simulink model "gm_gm_mpu6050_interface"  (R2017a)
settings: Solver=FixedStepDiscrete  StartTime=0.0  StopTime=inf  RelTol=1e-3  EnableMultiTasking=on
PostLoadFcn:
  | ChipSelect = 1;  % choose I2C comms
  | AddressAlt  = 0;  % use default address
  | 
  | if AddressAlt == 1
  | % b1101001 (pin AD0 is logic high).
  | SlvAddr = uint8(bin2dec('1101001'));  % ADDR ALT = 1
  | else
  | % b1101000 (pin AD0 is logic low)
  | SlvAddr = uint8(bin2dec('1101000'));  % ADDR ALT = 0
  | end
  | 
  | % 0x3B 59 ACCEL_XOUT[15:8]
  | % 0x3C 60 ACCEL_XOUT[7:0]
  | % 0x3D 61 ACCEL_YOUT[15:8]
  | % 0x3E 62 ACCEL_YOUT[7:0]
  | % 0x3F 63 ACCEL_ZOUT[15:8]
  | % 0x40 64 ACCEL_ZOUT[7:0]
  | 
  | AccelXRegAddr = uint8(hex2dec('3B'));
  | AccelYRegAddr = uint8(hex2dec('3D'));
  | AccelZRegAddr = uint8(hex2dec('3F'));
  | 
  | % 0x43 67 GYRO_XOUT[15:8]
  | % 0x44 68 GYRO_XOUT[7:0]
  | % 0x45 69 GYRO_YOUT[15:8]
  | % 0x46 70 GYRO_YOUT[7:0]
  | % 0x47 71 GYRO_ZOUT[15:8]
  | % 0x48 72 GYRO_ZOUT[7:0]
  | 
  | GyroXRegAddr = uint8(hex2dec('43'));
  | GyroYRegAddr = uint8(hex2dec('45'));
  | GyroZRegAddr = uint8(hex2dec('47'));
  | 
  | deviceAddr = fi(SlvAddr,0,7,0);
  | 
  | powerRegAddr = uint8(hex2dec('6B'));
  | powerRegData = bin2dec('10000001');
undefined symbols (not defined in the file or in its folder): AXI4, codertarget, gcbh, Lite
libraries: axiinterfacelib x9
settings Model: Creator=skuznick  LastModifiedBy=Nicoe Welch
settings SolverCC: EnableConcurrentExecution=on  ConcurrentTasks=on  PositivePriorityOrder=on
settings DataIOCC: SaveOutput=off  SaveTime=off
settings OptimizationCC: BlockReduction=off  ConditionallyExecuteInputs=off  PassReuseOutputArgsAs=Individual arguments  MaxStackSize=64
settings DebuggingCC: AlgebraicLoopMsg=error  InheritedTsInSrcMsg=none  SingleTaskRateTransMsg=error  ParameterTunabilityLossMsg=error
settings HardwareCC: ProdBitPerPointer=32  ProdBitPerSizeT=32  ProdBitPerPtrDiffT=32  ProdLargestAtomicInteger=Long  ProdLargestAtomicFloat=Double  ProdWordSize=32  ProdHWDeviceType=ARM Compatible->ARM Cortex  TargetEndianess=LittleEndian
settings SFSimCC: MATLABDynamicMemAlloc=off
settings RTWCC: SystemTargetFile=ert.tlc  HardwareBoard=ZedBoard  TLCOptions="-aInlineSetEventsForThisBaseRateFcn=TLC_FALSE -aSuppressMultiTaskScheduler=TLC_FALSE  -aRateBasedStepFcn=0"  TemplateMakefile=ert_default_tmf  Description=Embedded Coder  GenerateReport=on  Toolchain=Xilinx Software Development Kit (SDK)  IncludeHyperlinkInReport=on  LaunchReport=on  GenerateTraceInfo=on  GenerateTraceReport=on  GenerateTraceReportSl=on  GenerateTraceReportSf=on  GenerateTraceReportEml=on
settings CodeAppCC: ForceParamTrailComments=on  IgnoreCustomStorageClasses=off  OperatorAnnotations=on  SimulinkDataObjDesc=on  SFDataObjDesc=on  MATLABFcnDesc=on  InsertBlockDesc=on  MATLABSourceComments=on

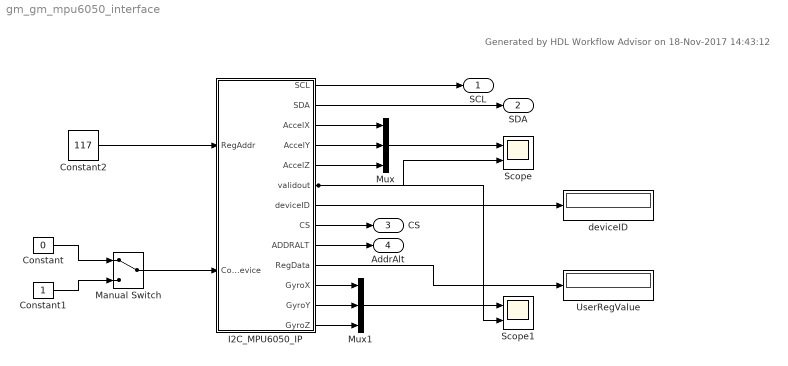
== system gm_gm_mpu6050_interface ==
  note: Generated by HDL Workflow Advisor on 18-Nov-2017 14:43:12
  Constant : Constant  Value=0  OutDataTypeStr=boolean  SampleTime=-1
  Constant1 : Constant  OutDataTypeStr=boolean  SampleTime=-1
  Constant2 : Constant  Value=117  OutDataTypeStr=uint8  SampleTime=-1
  I2C_MPU6050_IP : Subsystem  mask(AXI4-Lite/AXI4 Interface){}
      mask help:
      | This is an automatically generated subsystem block.
      | This contains the AXI interface blocks that communicate with the I2C_MPU60_ip IPCore generated from mpu6050/I2C_MPU6050_IP subsystem.
      mask Display: disp(sprintf('Xilinx Zynq \nAXI Interface'));
  Manual Switch : ManualSwitch
  Mux : Mux  Inputs=3
  Mux1 : Mux  Inputs=3
  Scope : Scope  NumInputPorts=2
  Scope1 : Scope  NumInputPorts=2
  UserRegValue : Display
  deviceID : Display
  SCL : Outport
  SDA : Outport  Port=2
  CS : Outport  Port=3
  AddrAlt : Outport  Port=4
  wires:
  I2C_MPU6050_IP/2(SDA) -> SDA/1
  I2C_MPU6050_IP/1(SCL) -> SCL/1
  I2C_MPU6050_IP/8(CS) -> CS/1
  I2C_MPU6050_IP/9(ADDRALT) -> AddrAlt/1
  I2C_MPU6050_IP/4(AccelY) -> Mux/2
  I2C_MPU6050_IP/3(AccelX) -> Mux/1
  I2C_MPU6050_IP/5(AccelZ) -> Mux/3
  I2C_MPU6050_IP/7(deviceID) -> deviceID/1
  I2C_MPU6050_IP/10(RegData) -> UserRegValue/1
  Mux/1 -> Scope/1
  Constant/1 -> Manual Switch/1
  Constant1/1 -> Manual Switch/2
  Manual Switch/1 -> I2C_MPU6050_IP/2(ConfigDevice)
  Constant2/1 -> I2C_MPU6050_IP/1(RegAddr)
  Mux1/1 -> Scope1/1
  I2C_MPU6050_IP/13(GyroZ) -> Mux1/3
  I2C_MPU6050_IP/11(GyroX) -> Mux1/1
  I2C_MPU6050_IP/12(GyroY) -> Mux1/2
  I2C_MPU6050_IP/6(validout) -> Scope/2, Scope1/2

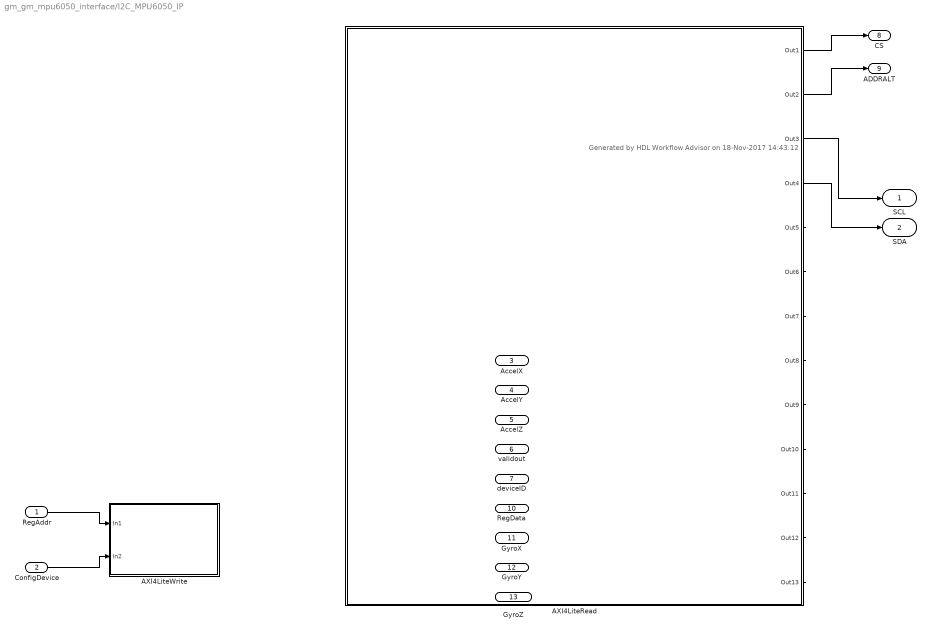
== system gm_gm_mpu6050_interface/I2C_MPU6050_IP ==
  note: Generated by HDL Workflow Advisor on 18-Nov-2017 14:43:12
  RegAddr : Inport  OutDataTypeStr=uint8  SampleTime=0.2
  ConfigDevice : Inport  Port=2  OutDataTypeStr=boolean  SampleTime=0.2
  AXI4LiteRead : Subsystem
  AXI4LiteWrite : Subsystem
  SCL : Outport
  SDA : Outport  Port=2
  AccelX : Outport  Port=3
  AccelY : Outport  Port=4
  AccelZ : Outport  Port=5
  validout : Outport  Port=6
  deviceID : Outport  Port=7
  CS : Outport  Port=8
  ADDRALT : Outport  Port=9
  RegData : Outport  Port=10
  GyroX : Outport  Port=11
  GyroY : Outport  Port=12
  GyroZ : Outport  Port=13
  wires:
  RegAddr/1 -> AXI4LiteWrite/1(In1)
  ConfigDevice/1 -> AXI4LiteWrite/2(In2)
  AXI4LiteRead/1(Out1) -> CS/1
  AXI4LiteRead/2(Out2) -> ADDRALT/1
  AXI4LiteRead/3(Out3) -> SCL/1
  AXI4LiteRead/4(Out4) -> SDA/1
  AXI4LiteRead/5(Out5) -> AccelX/1
  AXI4LiteRead/6(Out6) -> AccelY/1
  AXI4LiteRead/7(Out7) -> AccelZ/1
  AXI4LiteRead/8(Out8) -> validout/1
  AXI4LiteRead/9(Out9) -> deviceID/1
  AXI4LiteRead/10(Out10) -> RegData/1
  AXI4LiteRead/11(Out11) -> GyroX/1
  AXI4LiteRead/12(Out12) -> GyroY/1
  AXI4LiteRead/13(Out13) -> GyroZ/1

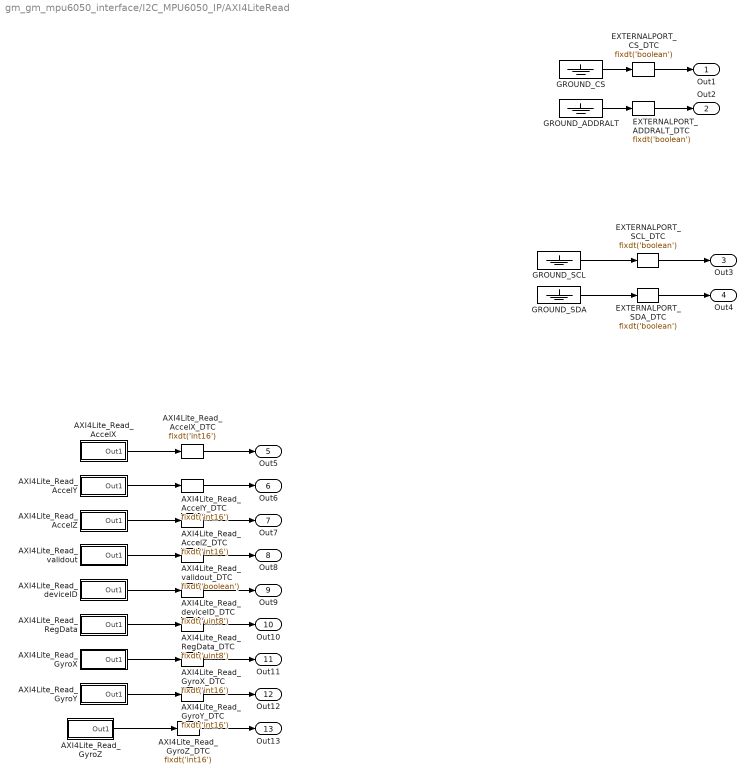
== system gm_gm_mpu6050_interface/I2C_MPU6050_IP/AXI4LiteRead ==
  AXI4Lite_Read_AccelX : Subsystem  InitFcn=codertarget.zynq.internal.registerAXIInterfaceBlocks(gcbh);  mask(AXI4-Interface Read){AXIInterfaceType='AXI4-Lite', DeviceName='/dev/mwipcore', RegisterOffset=hex2dec('104'), DataLength=1, DataType='uint32', SampleTime=-1, blockPlatform=ZYNQ, SimulateUsing=Interpreted Execution}
      mask prompts: AXIInterfaceType "AXI interface:"; DeviceName "Device name:"; RegisterOffset "Register offset:"; DataLength "Output vector size:"; DataType "Data type:"; SampleTime "Sample time:"; blockPlatform "Block Platform:"; SimulateUsing "Simulate Using:"
      mask help:
      | Read data from the IP core device using AXI interface.
      |
      | Set AXI interface parameter to 'AXI4-Lite' to read scalar data from the IP core register.
      |
      | Set AXI interface parameter to  'AXI4-Stream' to read vector data from DMA buffer. Use the Output vector size parameter to determine the number of samples read for each DMA transfer.
      mask init:
      | set_param(gcb, 'MaskDescription', DAStudio.message('zynq:utils:AXIReadMaskDisplay'));
      | set_param(gcb, 'MaskType','AXI4-Interface Read');
      | set_param(gcb, 'MaskHelp','eval(''slhelp([gcb,''''/AXI4-Interface Read''''])'');');
      | set_param(gcb, 'InitFcn', 'codertarget.zynq.internal.registerAXIInterfaceBlocks(gcbh);');
      mask Help: eval('slhelp([gcb,''/AXI4-Interface Read''])');
      mask Callback AXIInterfaceType:
      | if strcmpi(get_param(gcb, 'AXIInterfaceType'),'AXI4-Stream')
      |     set_param(gcb, 'MaskVisibilities',...
      |         {'on';'on';'off';'on';'on';'on';'off';'off'});
      | else
      |     set_param(gcb, 'MaskVisibilities',...
      |         {'on';'on';'on';'on';'on';'on';'off';'off'});
      | end
      mask TypeOptions SimulateUsing: Interpreted Execution | Code Generation
      mask Display:
      | text(0.50, 0.50, get_param([gcb,'/AXI4-Interface Read'], 'AXIInterfaceType'), ...
      |     'horizontalAlignment', 'center');
      | color('blue');
      | text(0.97, 0.87, get_param(gcb,'blockPlatform'), 'horizontalAlignment', 'right');
  AXI4Lite_Read_AccelX_DTC : DataTypeConversion  OutDataTypeStr=fixdt('int16')  ConvertRealWorld=Stored Integer (SI)
  AXI4Lite_Read_AccelY : Subsystem  InitFcn=codertarget.zynq.internal.registerAXIInterfaceBlocks(gcbh);  mask(AXI4-Interface Read){AXIInterfaceType='AXI4-Lite', DeviceName='/dev/mwipcore', RegisterOffset=hex2dec('108'), DataLength=1, DataType='uint32', SampleTime=-1, blockPlatform=ZYNQ, SimulateUsing=Interpreted Execution}
      mask prompts: AXIInterfaceType "AXI interface:"; DeviceName "Device name:"; RegisterOffset "Register offset:"; DataLength "Output vector size:"; DataType "Data type:"; SampleTime "Sample time:"; blockPlatform "Block Platform:"; SimulateUsing "Simulate Using:"
      mask help:
      | Read data from the IP core device using AXI interface.
      |
      | Set AXI interface parameter to 'AXI4-Lite' to read scalar data from the IP core register.
      |
      | Set AXI interface parameter to  'AXI4-Stream' to read vector data from DMA buffer. Use the Output vector size parameter to determine the number of samples read for each DMA transfer.
      mask init: same as gm_gm_mpu6050_interface/I2C_MPU6050_IP/AXI4LiteRead/AXI4Lite_Read_AccelX
      mask Help: eval('slhelp([gcb,''/AXI4-Interface Read''])');
      mask Callback AXIInterfaceType:
      | if strcmpi(get_param(gcb, 'AXIInterfaceType'),'AXI4-Stream')
      |     set_param(gcb, 'MaskVisibilities',...
      |         {'on';'on';'off';'on';'on';'on';'off';'off'});
      | else
      |     set_param(gcb, 'MaskVisibilities',...
      |         {'on';'on';'on';'on';'on';'on';'off';'off'});
      | end
      mask TypeOptions SimulateUsing: Interpreted Execution | Code Generation
      mask Display:
      | text(0.50, 0.50, get_param([gcb,'/AXI4-Interface Read'], 'AXIInterfaceType'), ...
      |     'horizontalAlignment', 'center');
      | color('blue');
      | text(0.97, 0.87, get_param(gcb,'blockPlatform'), 'horizontalAlignment', 'right');
  AXI4Lite_Read_AccelY_DTC : DataTypeConversion  OutDataTypeStr=fixdt('int16')  ConvertRealWorld=Stored Integer (SI)
  AXI4Lite_Read_AccelZ : Subsystem  InitFcn=codertarget.zynq.internal.registerAXIInterfaceBlocks(gcbh);  mask(AXI4-Interface Read){AXIInterfaceType='AXI4-Lite', DeviceName='/dev/mwipcore', RegisterOffset=hex2dec('10C'), DataLength=1, DataType='uint32', SampleTime=-1, blockPlatform=ZYNQ, SimulateUsing=Interpreted Execution}
      mask prompts: AXIInterfaceType "AXI interface:"; DeviceName "Device name:"; RegisterOffset "Register offset:"; DataLength "Output vector size:"; DataType "Data type:"; SampleTime "Sample time:"; blockPlatform "Block Platform:"; SimulateUsing "Simulate Using:"
      mask help:
      | Read data from the IP core device using AXI interface.
      |
      | Set AXI interface parameter to 'AXI4-Lite' to read scalar data from the IP core register.
      |
      | Set AXI interface parameter to  'AXI4-Stream' to read vector data from DMA buffer. Use the Output vector size parameter to determine the number of samples read for each DMA transfer.
      mask init: same as gm_gm_mpu6050_interface/I2C_MPU6050_IP/AXI4LiteRead/AXI4Lite_Read_AccelX
      mask Help: eval('slhelp([gcb,''/AXI4-Interface Read''])');
      mask Callback AXIInterfaceType:
      | if strcmpi(get_param(gcb, 'AXIInterfaceType'),'AXI4-Stream')
      |     set_param(gcb, 'MaskVisibilities',...
      |         {'on';'on';'off';'on';'on';'on';'off';'off'});
      | else
      |     set_param(gcb, 'MaskVisibilities',...
      |         {'on';'on';'on';'on';'on';'on';'off';'off'});
      | end
      mask TypeOptions SimulateUsing: Interpreted Execution | Code Generation
      mask Display:
      | text(0.50, 0.50, get_param([gcb,'/AXI4-Interface Read'], 'AXIInterfaceType'), ...
      |     'horizontalAlignment', 'center');
      | color('blue');
      | text(0.97, 0.87, get_param(gcb,'blockPlatform'), 'horizontalAlignment', 'right');
  AXI4Lite_Read_AccelZ_DTC : DataTypeConversion  OutDataTypeStr=fixdt('int16')  ConvertRealWorld=Stored Integer (SI)
  AXI4Lite_Read_GyroX : Subsystem  InitFcn=codertarget.zynq.internal.registerAXIInterfaceBlocks(gcbh);  mask(AXI4-Interface Read){AXIInterfaceType='AXI4-Lite', DeviceName='/dev/mwipcore', RegisterOffset=hex2dec('120'), DataLength=1, DataType='uint32', SampleTime=-1, blockPlatform=ZYNQ, SimulateUsing=Interpreted Execution}
      mask prompts: AXIInterfaceType "AXI interface:"; DeviceName "Device name:"; RegisterOffset "Register offset:"; DataLength "Output vector size:"; DataType "Data type:"; SampleTime "Sample time:"; blockPlatform "Block Platform:"; SimulateUsing "Simulate Using:"
      mask help:
      | Read data from the IP core device using AXI interface.
      |
      | Set AXI interface parameter to 'AXI4-Lite' to read scalar data from the IP core register.
      |
      | Set AXI interface parameter to  'AXI4-Stream' to read vector data from DMA buffer. Use the Output vector size parameter to determine the number of samples read for each DMA transfer.
      mask init: same as gm_gm_mpu6050_interface/I2C_MPU6050_IP/AXI4LiteRead/AXI4Lite_Read_AccelX
      mask Help: eval('slhelp([gcb,''/AXI4-Interface Read''])');
      mask Callback AXIInterfaceType:
      | if strcmpi(get_param(gcb, 'AXIInterfaceType'),'AXI4-Stream')
      |     set_param(gcb, 'MaskVisibilities',...
      |         {'on';'on';'off';'on';'on';'on';'off';'off'});
      | else
      |     set_param(gcb, 'MaskVisibilities',...
      |         {'on';'on';'on';'on';'on';'on';'off';'off'});
      | end
      mask TypeOptions SimulateUsing: Interpreted Execution | Code Generation
      mask Display:
      | text(0.50, 0.50, get_param([gcb,'/AXI4-Interface Read'], 'AXIInterfaceType'), ...
      |     'horizontalAlignment', 'center');
      | color('blue');
      | text(0.97, 0.87, get_param(gcb,'blockPlatform'), 'horizontalAlignment', 'right');
  AXI4Lite_Read_GyroX_DTC : DataTypeConversion  OutDataTypeStr=fixdt('int16')  ConvertRealWorld=Stored Integer (SI)
  AXI4Lite_Read_GyroY : Subsystem  InitFcn=codertarget.zynq.internal.registerAXIInterfaceBlocks(gcbh);  mask(AXI4-Interface Read){AXIInterfaceType='AXI4-Lite', DeviceName='/dev/mwipcore', RegisterOffset=hex2dec('124'), DataLength=1, DataType='uint32', SampleTime=-1, blockPlatform=ZYNQ, SimulateUsing=Interpreted Execution}
      mask prompts: AXIInterfaceType "AXI interface:"; DeviceName "Device name:"; RegisterOffset "Register offset:"; DataLength "Output vector size:"; DataType "Data type:"; SampleTime "Sample time:"; blockPlatform "Block Platform:"; SimulateUsing "Simulate Using:"
      mask help:
      | Read data from the IP core device using AXI interface.
      |
      | Set AXI interface parameter to 'AXI4-Lite' to read scalar data from the IP core register.
      |
      | Set AXI interface parameter to  'AXI4-Stream' to read vector data from DMA buffer. Use the Output vector size parameter to determine the number of samples read for each DMA transfer.
      mask init: same as gm_gm_mpu6050_interface/I2C_MPU6050_IP/AXI4LiteRead/AXI4Lite_Read_AccelX
      mask Help: eval('slhelp([gcb,''/AXI4-Interface Read''])');
      mask Callback AXIInterfaceType:
      | if strcmpi(get_param(gcb, 'AXIInterfaceType'),'AXI4-Stream')
      |     set_param(gcb, 'MaskVisibilities',...
      |         {'on';'on';'off';'on';'on';'on';'off';'off'});
      | else
      |     set_param(gcb, 'MaskVisibilities',...
      |         {'on';'on';'on';'on';'on';'on';'off';'off'});
      | end
      mask TypeOptions SimulateUsing: Interpreted Execution | Code Generation
      mask Display:
      | text(0.50, 0.50, get_param([gcb,'/AXI4-Interface Read'], 'AXIInterfaceType'), ...
      |     'horizontalAlignment', 'center');
      | color('blue');
      | text(0.97, 0.87, get_param(gcb,'blockPlatform'), 'horizontalAlignment', 'right');
  AXI4Lite_Read_GyroY_DTC : DataTypeConversion  OutDataTypeStr=fixdt('int16')  ConvertRealWorld=Stored Integer (SI)
  AXI4Lite_Read_GyroZ : Subsystem  InitFcn=codertarget.zynq.internal.registerAXIInterfaceBlocks(gcbh);  mask(AXI4-Interface Read){AXIInterfaceType='AXI4-Lite', DeviceName='/dev/mwipcore', RegisterOffset=hex2dec('128'), DataLength=1, DataType='uint32', SampleTime=-1, blockPlatform=ZYNQ, SimulateUsing=Interpreted Execution}
      mask prompts: AXIInterfaceType "AXI interface:"; DeviceName "Device name:"; RegisterOffset "Register offset:"; DataLength "Output vector size:"; DataType "Data type:"; SampleTime "Sample time:"; blockPlatform "Block Platform:"; SimulateUsing "Simulate Using:"
      mask help:
      | Read data from the IP core device using AXI interface.
      |
      | Set AXI interface parameter to 'AXI4-Lite' to read scalar data from the IP core register.
      |
      | Set AXI interface parameter to  'AXI4-Stream' to read vector data from DMA buffer. Use the Output vector size parameter to determine the number of samples read for each DMA transfer.
      mask init: same as gm_gm_mpu6050_interface/I2C_MPU6050_IP/AXI4LiteRead/AXI4Lite_Read_AccelX
      mask Help: eval('slhelp([gcb,''/AXI4-Interface Read''])');
      mask Callback AXIInterfaceType:
      | if strcmpi(get_param(gcb, 'AXIInterfaceType'),'AXI4-Stream')
      |     set_param(gcb, 'MaskVisibilities',...
      |         {'on';'on';'off';'on';'on';'on';'off';'off'});
      | else
      |     set_param(gcb, 'MaskVisibilities',...
      |         {'on';'on';'on';'on';'on';'on';'off';'off'});
      | end
      mask TypeOptions SimulateUsing: Interpreted Execution | Code Generation
      mask Display:
      | text(0.50, 0.50, get_param([gcb,'/AXI4-Interface Read'], 'AXIInterfaceType'), ...
      |     'horizontalAlignment', 'center');
      | color('blue');
      | text(0.97, 0.87, get_param(gcb,'blockPlatform'), 'horizontalAlignment', 'right');
  AXI4Lite_Read_GyroZ_DTC : DataTypeConversion  OutDataTypeStr=fixdt('int16')  ConvertRealWorld=Stored Integer (SI)
  AXI4Lite_Read_RegData : Subsystem  InitFcn=codertarget.zynq.internal.registerAXIInterfaceBlocks(gcbh);  mask(AXI4-Interface Read){AXIInterfaceType='AXI4-Lite', DeviceName='/dev/mwipcore', RegisterOffset=hex2dec('11C'), DataLength=1, DataType='uint32', SampleTime=-1, blockPlatform=ZYNQ, SimulateUsing=Interpreted Execution}
      mask prompts: AXIInterfaceType "AXI interface:"; DeviceName "Device name:"; RegisterOffset "Register offset:"; DataLength "Output vector size:"; DataType "Data type:"; SampleTime "Sample time:"; blockPlatform "Block Platform:"; SimulateUsing "Simulate Using:"
      mask help:
      | Read data from the IP core device using AXI interface.
      |
      | Set AXI interface parameter to 'AXI4-Lite' to read scalar data from the IP core register.
      |
      | Set AXI interface parameter to  'AXI4-Stream' to read vector data from DMA buffer. Use the Output vector size parameter to determine the number of samples read for each DMA transfer.
      mask init: same as gm_gm_mpu6050_interface/I2C_MPU6050_IP/AXI4LiteRead/AXI4Lite_Read_AccelX
      mask Help: eval('slhelp([gcb,''/AXI4-Interface Read''])');
      mask Callback AXIInterfaceType:
      | if strcmpi(get_param(gcb, 'AXIInterfaceType'),'AXI4-Stream')
      |     set_param(gcb, 'MaskVisibilities',...
      |         {'on';'on';'off';'on';'on';'on';'off';'off'});
      | else
      |     set_param(gcb, 'MaskVisibilities',...
      |         {'on';'on';'on';'on';'on';'on';'off';'off'});
      | end
      mask TypeOptions SimulateUsing: Interpreted Execution | Code Generation
      mask Display:
      | text(0.50, 0.50, get_param([gcb,'/AXI4-Interface Read'], 'AXIInterfaceType'), ...
      |     'horizontalAlignment', 'center');
      | color('blue');
      | text(0.97, 0.87, get_param(gcb,'blockPlatform'), 'horizontalAlignment', 'right');
  AXI4Lite_Read_RegData_DTC : DataTypeConversion  OutDataTypeStr=fixdt('uint8')  ConvertRealWorld=Stored Integer (SI)
  AXI4Lite_Read_deviceID : Subsystem  InitFcn=codertarget.zynq.internal.registerAXIInterfaceBlocks(gcbh);  mask(AXI4-Interface Read){AXIInterfaceType='AXI4-Lite', DeviceName='/dev/mwipcore', RegisterOffset=hex2dec('118'), DataLength=1, DataType='uint32', SampleTime=-1, blockPlatform=ZYNQ, SimulateUsing=Interpreted Execution}
      mask prompts: AXIInterfaceType "AXI interface:"; DeviceName "Device name:"; RegisterOffset "Register offset:"; DataLength "Output vector size:"; DataType "Data type:"; SampleTime "Sample time:"; blockPlatform "Block Platform:"; SimulateUsing "Simulate Using:"
      mask help:
      | Read data from the IP core device using AXI interface.
      |
      | Set AXI interface parameter to 'AXI4-Lite' to read scalar data from the IP core register.
      |
      | Set AXI interface parameter to  'AXI4-Stream' to read vector data from DMA buffer. Use the Output vector size parameter to determine the number of samples read for each DMA transfer.
      mask init: same as gm_gm_mpu6050_interface/I2C_MPU6050_IP/AXI4LiteRead/AXI4Lite_Read_AccelX
      mask Help: eval('slhelp([gcb,''/AXI4-Interface Read''])');
      mask Callback AXIInterfaceType:
      | if strcmpi(get_param(gcb, 'AXIInterfaceType'),'AXI4-Stream')
      |     set_param(gcb, 'MaskVisibilities',...
      |         {'on';'on';'off';'on';'on';'on';'off';'off'});
      | else
      |     set_param(gcb, 'MaskVisibilities',...
      |         {'on';'on';'on';'on';'on';'on';'off';'off'});
      | end
      mask TypeOptions SimulateUsing: Interpreted Execution | Code Generation
      mask Display:
      | text(0.50, 0.50, get_param([gcb,'/AXI4-Interface Read'], 'AXIInterfaceType'), ...
      |     'horizontalAlignment', 'center');
      | color('blue');
      | text(0.97, 0.87, get_param(gcb,'blockPlatform'), 'horizontalAlignment', 'right');
  AXI4Lite_Read_deviceID_DTC : DataTypeConversion  OutDataTypeStr=fixdt('uint8')  ConvertRealWorld=Stored Integer (SI)
  AXI4Lite_Read_validout : Subsystem  InitFcn=codertarget.zynq.internal.registerAXIInterfaceBlocks(gcbh);  mask(AXI4-Interface Read){AXIInterfaceType='AXI4-Lite', DeviceName='/dev/mwipcore', RegisterOffset=hex2dec('110'), DataLength=1, DataType='uint32', SampleTime=-1, blockPlatform=ZYNQ, SimulateUsing=Interpreted Execution}
      mask prompts: AXIInterfaceType "AXI interface:"; DeviceName "Device name:"; RegisterOffset "Register offset:"; DataLength "Output vector size:"; DataType "Data type:"; SampleTime "Sample time:"; blockPlatform "Block Platform:"; SimulateUsing "Simulate Using:"
      mask help:
      | Read data from the IP core device using AXI interface.
      |
      | Set AXI interface parameter to 'AXI4-Lite' to read scalar data from the IP core register.
      |
      | Set AXI interface parameter to  'AXI4-Stream' to read vector data from DMA buffer. Use the Output vector size parameter to determine the number of samples read for each DMA transfer.
      mask init: same as gm_gm_mpu6050_interface/I2C_MPU6050_IP/AXI4LiteRead/AXI4Lite_Read_AccelX
      mask Help: eval('slhelp([gcb,''/AXI4-Interface Read''])');
      mask Callback AXIInterfaceType:
      | if strcmpi(get_param(gcb, 'AXIInterfaceType'),'AXI4-Stream')
      |     set_param(gcb, 'MaskVisibilities',...
      |         {'on';'on';'off';'on';'on';'on';'off';'off'});
      | else
      |     set_param(gcb, 'MaskVisibilities',...
      |         {'on';'on';'on';'on';'on';'on';'off';'off'});
      | end
      mask TypeOptions SimulateUsing: Interpreted Execution | Code Generation
      mask Display:
      | text(0.50, 0.50, get_param([gcb,'/AXI4-Interface Read'], 'AXIInterfaceType'), ...
      |     'horizontalAlignment', 'center');
      | color('blue');
      | text(0.97, 0.87, get_param(gcb,'blockPlatform'), 'horizontalAlignment', 'right');
  AXI4Lite_Read_validout_DTC : DataTypeConversion  OutDataTypeStr=fixdt('boolean')  ConvertRealWorld=Stored Integer (SI)
  EXTERNALPORT_ADDRALT_DTC : DataTypeConversion  OutDataTypeStr=fixdt('boolean')
  EXTERNALPORT_CS_DTC : DataTypeConversion  OutDataTypeStr=fixdt('boolean')
  EXTERNALPORT_SCL_DTC : DataTypeConversion  OutDataTypeStr=fixdt('boolean')
  EXTERNALPORT_SDA_DTC : DataTypeConversion  OutDataTypeStr=fixdt('boolean')
  GROUND_ADDRALT : Ground
  GROUND_CS : Ground
  GROUND_SCL : Ground
  GROUND_SDA : Ground
  Out1 : Outport
  Out2 : Outport  Port=2
  Out3 : Outport  Port=3
  Out4 : Outport  Port=4
  Out5 : Outport  Port=5
  Out6 : Outport  Port=6
  Out7 : Outport  Port=7
  Out8 : Outport  Port=8
  Out9 : Outport  Port=9
  Out10 : Outport  Port=10
  Out11 : Outport  Port=11
  Out12 : Outport  Port=12
  Out13 : Outport  Port=13
  wires:
  AXI4Lite_Read_AccelX/1(Out1) -> AXI4Lite_Read_AccelX_DTC/1
  AXI4Lite_Read_AccelX_DTC/1 -> Out5/1
  AXI4Lite_Read_AccelY/1(Out1) -> AXI4Lite_Read_AccelY_DTC/1
  AXI4Lite_Read_AccelY_DTC/1 -> Out6/1
  AXI4Lite_Read_AccelZ/1(Out1) -> AXI4Lite_Read_AccelZ_DTC/1
  AXI4Lite_Read_AccelZ_DTC/1 -> Out7/1
  AXI4Lite_Read_GyroX/1(Out1) -> AXI4Lite_Read_GyroX_DTC/1
  AXI4Lite_Read_GyroX_DTC/1 -> Out11/1
  AXI4Lite_Read_GyroY/1(Out1) -> AXI4Lite_Read_GyroY_DTC/1
  AXI4Lite_Read_GyroY_DTC/1 -> Out12/1
  AXI4Lite_Read_GyroZ/1(Out1) -> AXI4Lite_Read_GyroZ_DTC/1
  AXI4Lite_Read_GyroZ_DTC/1 -> Out13/1
  AXI4Lite_Read_RegData/1(Out1) -> AXI4Lite_Read_RegData_DTC/1
  AXI4Lite_Read_RegData_DTC/1 -> Out10/1
  AXI4Lite_Read_deviceID/1(Out1) -> AXI4Lite_Read_deviceID_DTC/1
  AXI4Lite_Read_deviceID_DTC/1 -> Out9/1
  AXI4Lite_Read_validout/1(Out1) -> AXI4Lite_Read_validout_DTC/1
  AXI4Lite_Read_validout_DTC/1 -> Out8/1
  EXTERNALPORT_ADDRALT_DTC/1 -> Out2/1
  EXTERNALPORT_CS_DTC/1 -> Out1/1
  EXTERNALPORT_SCL_DTC/1 -> Out3/1
  EXTERNALPORT_SDA_DTC/1 -> Out4/1
  GROUND_ADDRALT/1 -> EXTERNALPORT_ADDRALT_DTC/1
  GROUND_CS/1 -> EXTERNALPORT_CS_DTC/1
  GROUND_SCL/1 -> EXTERNALPORT_SCL_DTC/1
  GROUND_SDA/1 -> EXTERNALPORT_SDA_DTC/1

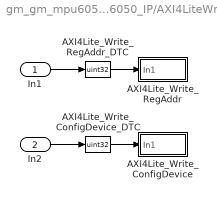
== system gm_gm_mpu6050_interface/I2C_MPU6050_IP/AXI4LiteWrite ==
  In1 : Inport  SampleTime=0.2
  In2 : Inport  Port=2  SampleTime=0.2
  AXI4Lite_Write_ConfigDevice : Subsystem  InitFcn=codertarget.zynq.internal.registerAXIInterfaceBlocks(gcbh);  mask(AXI4-Interface Write){AXIInterfaceType='AXI4-Lite', DeviceName='/dev/mwipcore', RegisterOffset=hex2dec('100'), blockPlatform=ZYNQ, SimulateUsing=Interpreted execution}
      mask prompts: AXIInterfaceType "AXI interface:"; DeviceName "Device name:"; RegisterOffset "Register offset:"; blockPlatform "Block platform:"; SimulateUsing "Simulate using:"
      mask help:
      | Write data to the IP core device using AXI interface.
      |
      | Set AXI interface parameter to 'AXI4-Lite' to write scalar data to the IP core register.
      |
      | Set AXI interface parameter to  'AXI4-Stream' to write vector data to DMA buffer.
      mask init:
      | set_param(gcb, 'MaskDescription', DAStudio.message('zynq:utils:AXIWriteMaskDisplay'));
      | set_param(gcb, 'MaskType','AXI4-Interface Write');
      | set_param(gcb, 'MaskHelp','eval(''slhelp([gcb,''''/AXI4-Interface Write''''])'');');
      | set_param(gcb, 'InitFcn', 'codertarget.zynq.internal.registerAXIInterfaceBlocks(gcbh);')
      mask Help: eval('slhelp([gcb,''/AXI4-Interface Write''])');
      mask Callback AXIInterfaceType:
      | if strcmpi(get_param(gcb, 'AXIInterfaceType'),'AXI4-Stream')
      |     set_param(gcb, 'MaskVisibilities',...
      |         {'on';'on';'off';'off';'off'});
      | else
      |     set_param(gcb, 'MaskVisibilities',...
      |         {'on';'on';'on';'off';'off'});
      | end
      mask TypeOptions SimulateUsing: Interpreted execution | Code generation
      mask Display:
      | text(0.50, 0.50, get_param([gcb,'/AXI4-Interface Write'], 'AXIInterfaceType'), ...
      |     'horizontalAlignment', 'center');
      | color('blue');
      | text(0.97, 0.87, get_param(gcb,'blockPlatform'), 'horizontalAlignment', 'right');
  AXI4Lite_Write_ConfigDevice_DTC : DataTypeConversion  OutDataTypeStr=uint32  ConvertRealWorld=Stored Integer (SI)
  AXI4Lite_Write_RegAddr : Subsystem  InitFcn=codertarget.zynq.internal.registerAXIInterfaceBlocks(gcbh);  mask(AXI4-Interface Write){AXIInterfaceType='AXI4-Lite', DeviceName='/dev/mwipcore', RegisterOffset=hex2dec('114'), blockPlatform=ZYNQ, SimulateUsing=Interpreted execution}
      mask prompts: AXIInterfaceType "AXI interface:"; DeviceName "Device name:"; RegisterOffset "Register offset:"; blockPlatform "Block platform:"; SimulateUsing "Simulate using:"
      mask help:
      | Write data to the IP core device using AXI interface.
      |
      | Set AXI interface parameter to 'AXI4-Lite' to write scalar data to the IP core register.
      |
      | Set AXI interface parameter to  'AXI4-Stream' to write vector data to DMA buffer.
      mask init: same as gm_gm_mpu6050_interface/I2C_MPU6050_IP/AXI4LiteWrite/AXI4Lite_Write_ConfigDevice
      mask Help: eval('slhelp([gcb,''/AXI4-Interface Write''])');
      mask Callback AXIInterfaceType:
      | if strcmpi(get_param(gcb, 'AXIInterfaceType'),'AXI4-Stream')
      |     set_param(gcb, 'MaskVisibilities',...
      |         {'on';'on';'off';'off';'off'});
      | else
      |     set_param(gcb, 'MaskVisibilities',...
      |         {'on';'on';'on';'off';'off'});
      | end
      mask TypeOptions SimulateUsing: Interpreted execution | Code generation
      mask Display:
      | text(0.50, 0.50, get_param([gcb,'/AXI4-Interface Write'], 'AXIInterfaceType'), ...
      |     'horizontalAlignment', 'center');
      | color('blue');
      | text(0.97, 0.87, get_param(gcb,'blockPlatform'), 'horizontalAlignment', 'right');
  AXI4Lite_Write_RegAddr_DTC : DataTypeConversion  OutDataTypeStr=uint32  ConvertRealWorld=Stored Integer (SI)
  wires:
  In1/1 -> AXI4Lite_Write_RegAddr_DTC/1
  In2/1 -> AXI4Lite_Write_ConfigDevice_DTC/1
  AXI4Lite_Write_ConfigDevice_DTC/1 -> AXI4Lite_Write_ConfigDevice/1(In1)
  AXI4Lite_Write_RegAddr_DTC/1 -> AXI4Lite_Write_RegAddr/1(In1)

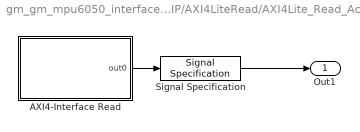
== system gm_gm_mpu6050_interface/I2C_MPU6050_IP/AXI4LiteRead/AXI4Lite_Read_AccelX ==
  AXI4-Interface Read : Subsystem
  Signal Specification : SignalSpecification
  Out1 : Outport
  wires:
  AXI4-Interface Read/1(out0) -> Signal Specification/1
  Signal Specification/1 -> Out1/1

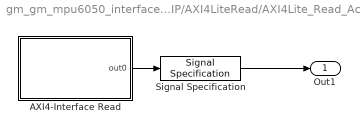
== system gm_gm_mpu6050_interface/I2C_MPU6050_IP/AXI4LiteRead/AXI4Lite_Read_AccelY ==
  AXI4-Interface Read : Subsystem
  Signal Specification : SignalSpecification
  Out1 : Outport
  wires:
  AXI4-Interface Read/1(out0) -> Signal Specification/1
  Signal Specification/1 -> Out1/1

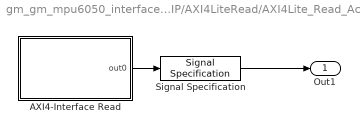
== system gm_gm_mpu6050_interface/I2C_MPU6050_IP/AXI4LiteRead/AXI4Lite_Read_AccelZ ==
  AXI4-Interface Read : Subsystem
  Signal Specification : SignalSpecification
  Out1 : Outport
  wires:
  AXI4-Interface Read/1(out0) -> Signal Specification/1
  Signal Specification/1 -> Out1/1

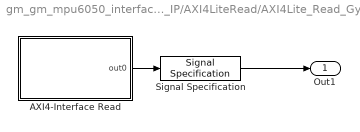
== system gm_gm_mpu6050_interface/I2C_MPU6050_IP/AXI4LiteRead/AXI4Lite_Read_GyroX ==
  AXI4-Interface Read : Subsystem
  Signal Specification : SignalSpecification
  Out1 : Outport
  wires:
  AXI4-Interface Read/1(out0) -> Signal Specification/1
  Signal Specification/1 -> Out1/1

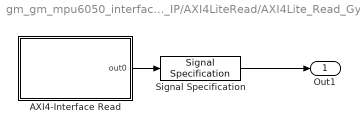
== system gm_gm_mpu6050_interface/I2C_MPU6050_IP/AXI4LiteRead/AXI4Lite_Read_GyroY ==
  AXI4-Interface Read : Subsystem
  Signal Specification : SignalSpecification
  Out1 : Outport
  wires:
  AXI4-Interface Read/1(out0) -> Signal Specification/1
  Signal Specification/1 -> Out1/1

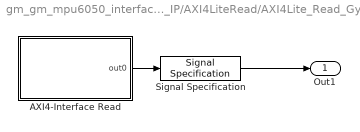
== system gm_gm_mpu6050_interface/I2C_MPU6050_IP/AXI4LiteRead/AXI4Lite_Read_GyroZ ==
  AXI4-Interface Read : Subsystem
  Signal Specification : SignalSpecification
  Out1 : Outport
  wires:
  AXI4-Interface Read/1(out0) -> Signal Specification/1
  Signal Specification/1 -> Out1/1

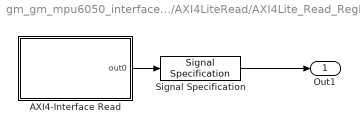
== system gm_gm_mpu6050_interface/I2C_MPU6050_IP/AXI4LiteRead/AXI4Lite_Read_RegData ==
  AXI4-Interface Read : Subsystem
  Signal Specification : SignalSpecification
  Out1 : Outport
  wires:
  AXI4-Interface Read/1(out0) -> Signal Specification/1
  Signal Specification/1 -> Out1/1

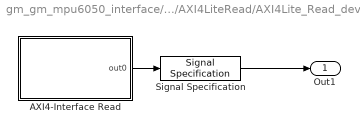
== system gm_gm_mpu6050_interface/I2C_MPU6050_IP/AXI4LiteRead/AXI4Lite_Read_deviceID ==
  AXI4-Interface Read : Subsystem
  Signal Specification : SignalSpecification
  Out1 : Outport
  wires:
  AXI4-Interface Read/1(out0) -> Signal Specification/1
  Signal Specification/1 -> Out1/1

== system gm_gm_mpu6050_interface/I2C_MPU6050_IP/AXI4LiteRead/AXI4Lite_Read_validout ==
  AXI4-Interface Read : Subsystem
  Signal Specification : SignalSpecification
  Out1 : Outport
  wires:
  AXI4-Interface Read/1(out0) -> Signal Specification/1
  Signal Specification/1 -> Out1/1

== system gm_gm_mpu6050_interface/I2C_MPU6050_IP/AXI4LiteWrite/AXI4Lite_Write_ConfigDevice ==
  In1 : Inport  OutDataTypeStr=uint32  SampleTime=0.2
  AXI4-Interface Write : Subsystem
  Signal Specification : SignalSpecification
  wires:
  In1/1 -> Signal Specification/1
  Signal Specification/1 -> AXI4-Interface Write/1(in0)

== system gm_gm_mpu6050_interface/I2C_MPU6050_IP/AXI4LiteWrite/AXI4Lite_Write_RegAddr ==
  In1 : Inport  OutDataTypeStr=uint32  SampleTime=0.2
  AXI4-Interface Write : Subsystem
  Signal Specification : SignalSpecification
  wires:
  In1/1 -> Signal Specification/1
  Signal Specification/1 -> AXI4-Interface Write/1(in0)

== system gm_gm_mpu6050_interface/I2C_MPU6050_IP/AXI4LiteRead/AXI4Lite_Read_AccelX/AXI4-Interface Read ==
  AXI4-Interface Read : axiinterfacelib/AXI4-Interface Read/AXI4-Interface Read  AXIInterfaceType=AXI4-Lite  DeviceName=/dev/mwipcore  RegisterOffset=RegisterOffset  DataType=uint32  DataLength=DataLength  SampleTime=SampleTime
      settings: SourceProductName=Embedded Coder Support Package for Xilinx Zynq-7000 Platform  SourceProductBaseCode=ECZYNQ7000
  out0 : Outport
  wires:
  AXI4-Interface Read/1 -> out0/1

== system gm_gm_mpu6050_interface/I2C_MPU6050_IP/AXI4LiteRead/AXI4Lite_Read_AccelY/AXI4-Interface Read ==
  AXI4-Interface Read : axiinterfacelib/AXI4-Interface Read/AXI4-Interface Read  AXIInterfaceType=AXI4-Lite  DeviceName=/dev/mwipcore  RegisterOffset=RegisterOffset  DataType=uint32  DataLength=DataLength  SampleTime=SampleTime
      settings: SourceProductName=Embedded Coder Support Package for Xilinx Zynq-7000 Platform  SourceProductBaseCode=ECZYNQ7000
  out0 : Outport
  wires:
  AXI4-Interface Read/1 -> out0/1

== system gm_gm_mpu6050_interface/I2C_MPU6050_IP/AXI4LiteRead/AXI4Lite_Read_AccelZ/AXI4-Interface Read ==
  AXI4-Interface Read : axiinterfacelib/AXI4-Interface Read/AXI4-Interface Read  AXIInterfaceType=AXI4-Lite  DeviceName=/dev/mwipcore  RegisterOffset=RegisterOffset  DataType=uint32  DataLength=DataLength  SampleTime=SampleTime
      settings: SourceProductName=Embedded Coder Support Package for Xilinx Zynq-7000 Platform  SourceProductBaseCode=ECZYNQ7000
  out0 : Outport
  wires:
  AXI4-Interface Read/1 -> out0/1

== system gm_gm_mpu6050_interface/I2C_MPU6050_IP/AXI4LiteRead/AXI4Lite_Read_GyroX/AXI4-Interface Read ==
  AXI4-Interface Read : axiinterfacelib/AXI4-Interface Read/AXI4-Interface Read  AXIInterfaceType=AXI4-Lite  DeviceName=/dev/mwipcore  RegisterOffset=RegisterOffset  DataType=uint32  DataLength=DataLength  SampleTime=SampleTime
      settings: SourceProductName=Embedded Coder Support Package for Xilinx Zynq-7000 Platform  SourceProductBaseCode=ECZYNQ7000
  out0 : Outport
  wires:
  AXI4-Interface Read/1 -> out0/1

== system gm_gm_mpu6050_interface/I2C_MPU6050_IP/AXI4LiteRead/AXI4Lite_Read_GyroY/AXI4-Interface Read ==
  AXI4-Interface Read : axiinterfacelib/AXI4-Interface Read/AXI4-Interface Read  AXIInterfaceType=AXI4-Lite  DeviceName=/dev/mwipcore  RegisterOffset=RegisterOffset  DataType=uint32  DataLength=DataLength  SampleTime=SampleTime
      settings: SourceProductName=Embedded Coder Support Package for Xilinx Zynq-7000 Platform  SourceProductBaseCode=ECZYNQ7000
  out0 : Outport
  wires:
  AXI4-Interface Read/1 -> out0/1

== system gm_gm_mpu6050_interface/I2C_MPU6050_IP/AXI4LiteRead/AXI4Lite_Read_GyroZ/AXI4-Interface Read ==
  AXI4-Interface Read : axiinterfacelib/AXI4-Interface Read/AXI4-Interface Read  AXIInterfaceType=AXI4-Lite  DeviceName=/dev/mwipcore  RegisterOffset=RegisterOffset  DataType=uint32  DataLength=DataLength  SampleTime=SampleTime
      settings: SourceProductName=Embedded Coder Support Package for Xilinx Zynq-7000 Platform  SourceProductBaseCode=ECZYNQ7000
  out0 : Outport
  wires:
  AXI4-Interface Read/1 -> out0/1

== system gm_gm_mpu6050_interface/I2C_MPU6050_IP/AXI4LiteRead/AXI4Lite_Read_RegData/AXI4-Interface Read ==
  AXI4-Interface Read : axiinterfacelib/AXI4-Interface Read/AXI4-Interface Read  AXIInterfaceType=AXI4-Lite  DeviceName=/dev/mwipcore  RegisterOffset=RegisterOffset  DataType=uint32  DataLength=DataLength  SampleTime=SampleTime
      settings: SourceProductName=Embedded Coder Support Package for Xilinx Zynq-7000 Platform  SourceProductBaseCode=ECZYNQ7000
  out0 : Outport
  wires:
  AXI4-Interface Read/1 -> out0/1

== system gm_gm_mpu6050_interface/I2C_MPU6050_IP/AXI4LiteRead/AXI4Lite_Read_deviceID/AXI4-Interface Read ==
  AXI4-Interface Read : axiinterfacelib/AXI4-Interface Read/AXI4-Interface Read  AXIInterfaceType=AXI4-Lite  DeviceName=/dev/mwipcore  RegisterOffset=RegisterOffset  DataType=uint32  DataLength=DataLength  SampleTime=SampleTime
      settings: SourceProductName=Embedded Coder Support Package for Xilinx Zynq-7000 Platform  SourceProductBaseCode=ECZYNQ7000
  out0 : Outport
  wires:
  AXI4-Interface Read/1 -> out0/1

== system gm_gm_mpu6050_interface/I2C_MPU6050_IP/AXI4LiteRead/AXI4Lite_Read_validout/AXI4-Interface Read ==
  AXI4-Interface Read : axiinterfacelib/AXI4-Interface Read/AXI4-Interface Read  AXIInterfaceType=AXI4-Lite  DeviceName=/dev/mwipcore  RegisterOffset=RegisterOffset  DataType=uint32  DataLength=DataLength  SampleTime=SampleTime
      settings: SourceProductName=Embedded Coder Support Package for Xilinx Zynq-7000 Platform  SourceProductBaseCode=ECZYNQ7000
  out0 : Outport
  wires:
  AXI4-Interface Read/1 -> out0/1

== system gm_gm_mpu6050_interface/I2C_MPU6050_IP/AXI4LiteWrite/AXI4Lite_Write_ConfigDevice/AXI4-Interface Write ==
  in0 : Inport  OutDataTypeStr=uint32  SampleTime=0.2

== system gm_gm_mpu6050_interface/I2C_MPU6050_IP/AXI4LiteWrite/AXI4Lite_Write_RegAddr/AXI4-Interface Write ==
  in0 : Inport  OutDataTypeStr=uint32  SampleTime=0.2
